simulink model "liti3"  (Simulink 5.0)
settings: Solver=ode45  SolverMode=SingleTasking  StartTime=0.0  StopTime=10  FixedStep=0.02  RelTol=1e-3
libraries: cstblocks x2
settings Model: LastModifiedBy=Administrator

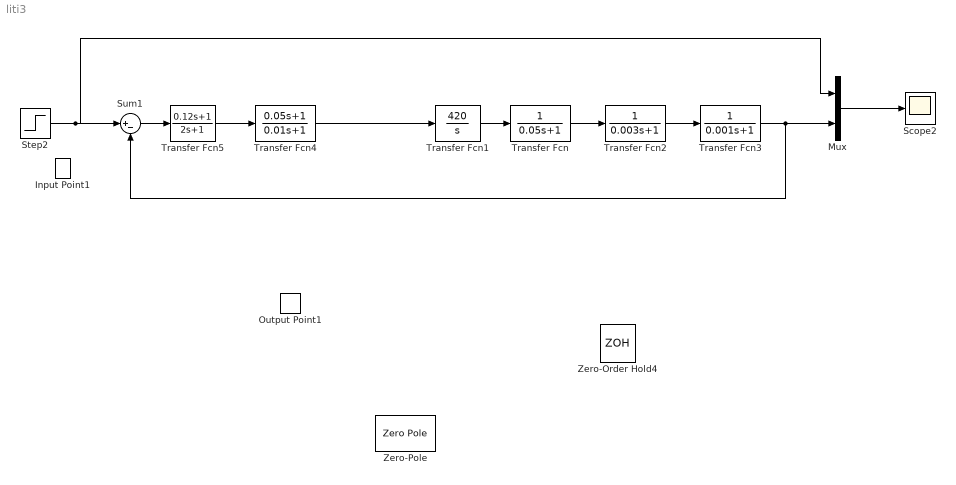
== system liti3 ==
  Input Point1 : cstblocks/Input Point
  Mux : Mux  Inputs=2
  Output Point1 : cstblocks/Output Point
  Scope2 : Scope
      settings: YMin=-3.5  YMax=1  MaxDataPoints=500000
  Step2 : Step  Time=0  SampleTime=0
  Sum1 : Sum  Inputs=|+-  SaturateOnIntegerOverflow=on
  Transfer Fcn : TransferFcn  Denominator=[0.05 1]
  Transfer Fcn1 : TransferFcn  Numerator=[420]  Denominator=[1 0]
  Transfer Fcn2 : TransferFcn  Denominator=[0.003 1]
  Transfer Fcn3 : TransferFcn  Denominator=[0.001 1]
  Transfer Fcn4 : TransferFcn  Numerator=[0.05 1]  Denominator=[0.01 1]
  Transfer Fcn5 : TransferFcn  Numerator=[0.12 1]  Denominator=[2 1]
  Zero-Order Hold4 : ZeroOrderHold  SampleTime=0.02
  Zero-Pole : ZeroPole  Zeros=[]  Poles=[0 -2]  Gain=[4]
  wires:
  Mux/1 -> Scope2/1
  Transfer Fcn/1 -> Transfer Fcn2/1
  Step2/1 -> Mux/1, Sum1/1
  Transfer Fcn1/1 -> Transfer Fcn/1
  Transfer Fcn2/1 -> Transfer Fcn3/1
  Transfer Fcn3/1 -> Mux/2, Sum1/2
  Transfer Fcn4/1 -> Transfer Fcn1/1
  Transfer Fcn5/1 -> Transfer Fcn4/1
  Sum1/1 -> Transfer Fcn5/1
